simulink model "mpc_controller1"  (R2024a)
settings: Solver=VariableStepAuto  StartTime=0.0  StopTime=12  RelTol=1e-3
InitFcn:
  | % MPC Tuning:
  | % Control Voltage was low, settling of the state variables is slow.
  | % Sol1: Decrease mpc1.Weights.MVRate (the penalty on voltage be cheaper)
  | % Sol2: Increase the weights penalty (same, more expensive error)
  | % Sol3: Initial conditions should not be near the constraints.
  | 
  | % For 1000 Hz sample rate with sensors, and 100 Hz sample rate MPC, the
  | % 200 long predict and 10 long control horizon should be enough,
  | % the system can't change faster.
  | 
  | % MPC tuning params
  | horizonNum = 200;
  | controlHorizon = 10;
  | 
  | MVWeight = 0;
  | MVRateWeight = 0.1;
  | stateVariableWeights = [0 0 10 0 0 0];
  | ECR = 10;
  | 
  | % MPC Constraints
  | x_m = 0.1;
  | x_dot_m = 2;
  | phi_m = 0.2;
  | phi_dot_m = 5;
  | i_m = 2;
  | w_m = 100;
  | 
  | % Init model
  | dt = 1/1000;
  | model_dt = dt;
  | 
  | A_aug =[ 0    0.0010         0         0         0         0;
  |          0         0   -0.0010         0    0.8250         0;
  |          0         0         0    0.0010         0         0;
  |          0         0    0.0473         0   -3.6197         0;
  |          0         0         0         0   -0.0591   -0.0022;
  |          0         0         0         0    0.3401   -0.0031];
  | B_aug = [0
  |          0;
  |          0;
  |          0;
  |        200;
  |          0];
  | C_aug = [    1     0     0     0     0     0;
  |              0     0     1     0     0     0];
  | D_aug = [0;0];
  | 
  | % Discretize System - for the augmented system
  | sysd = c2d(ss(A_aug, B_aug, C_aug, 0), dt);
  | Ad_aug = sysd.A;
  | Bd_aug = sysd.B;
  | Cd_aug = sysd.C;
  | 
  | % MPC
  | mpc_dt = 1/100;
  | robSys_mpc = c2d(ss(A_aug, B_aug, eye(6), zeros(6,1)), mpc_dt);
  | %% create MPC controller object with sample time
  | mpc1 = mpc(robSys_mpc, mpc_dt);
  | %% specify prediction horizon
  | mpc1.PredictionHorizon = horizonNum;
  | %% specify control horizon
  | mpc1.ControlHorizon = controlHorizon;
  | %% specify nominal values for inputs and outputs
  | mpc1.Model.Nominal.U = 0;
  | mpc1.Model.Nominal.Y = [0;0;0;0;0;0];
  | %% specify constraints for MV and MV Rate
  | mpc1.MV(1).Min = -12;
  | mpc1.MV(1).Max = 12;
  | %% specify constraints for OV
  | mpc1.OV(1).Min = -x_m;
  | mpc1.OV(1).Max = x_m;
  | mpc1.OV(2).Min = -x_dot_m;
  | mpc1.OV(2).Max = x_dot_m;
  | mpc1.OV(3).Min = -phi_m;
  | mpc1.OV(3).Max = phi_m;
  | mpc1.OV(4).Min = -phi_dot_m;
  | mpc1.OV(4).Max = phi_dot_m;
  | mpc1.OV(5).Min = -i_m;
  | mpc1.OV(5).Max = i_m;
  | mpc1.OV(6).Min = -w_m;
  | mpc1.OV(6).Max = w_m;
  | %% specify overall adjustment factor applied to weights
  | beta = 6.821;
  | %% specify weights
  | mpc1.Weights.MV = MVWeight;
  | mpc1.Weights.MVRate = MVRateWeight;
  | mpc1.Weights.OV = stateVariableWeights;
  | mpc1.Weights.ECR = ECR;
  | %% specify overall adjustment factor applied to estimation model gains
  | alpha = 4.1687;
  | %% adjust default output disturbance model gains
  | setoutdist(mpc1, 'model', getoutdist(mpc1)*alpha);
  | %% adjust default measurement noise model gains
  | mpc1.Model.Noise = mpc1.Model.Noise/alpha;
  | %% specify simulation options
  | options = mpcsimopt();
  | options.RefLookAhead = 'off';
  | options.MDLookAhead = 'off';
  | options.Constraints = 'on';
  | options.OpenLoop = 'off';
undefined symbols (not defined in the file or in its folder): Discrete, Time
libraries: ctrlSharedLib x1, mpclib x1
settings Model: Creator=Peter  LastModifiedBy=Peter

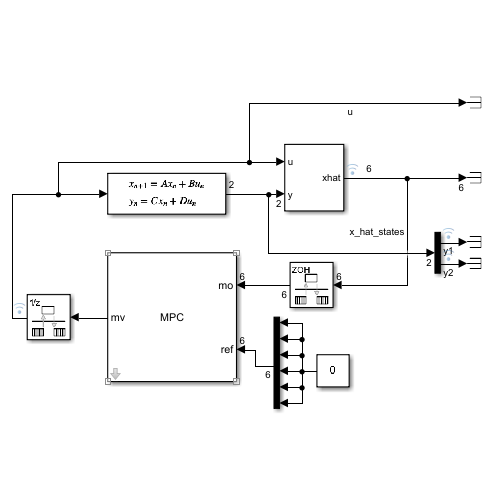
[thumbnail: Simulink's stored preview of the top-level diagram]
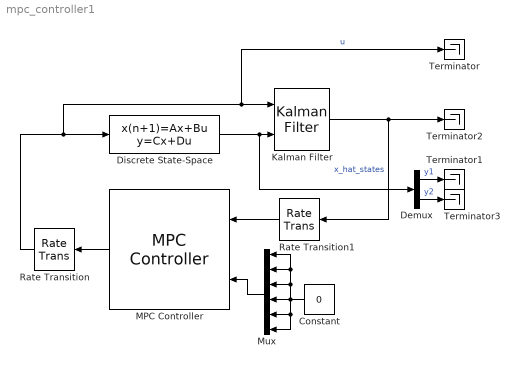
== system mpc_controller1 ==
  Constant : Constant  Value=0
  Demux : Demux  Outputs=2
  Discrete State-Space : DiscreteStateSpace  A=Ad_aug  B=Bd_aug  C=Cd_aug  D=[0;0]  InitialCondition=[0;0;0.05;0;0;0]  SampleTime=model_dt
  Kalman Filter : ctrlSharedLib/Kalman Filter  TimeDomain=Discrete-Time  UseCurrentEstimator=on  ModelSource=Individual A, B, C, D matrices  ModelSourceVariable=ss(0.95,1,1,0,1)  A=Ad_aug  B=Bd_aug  C=Cd_aug  D=[0;0]  NumberOfStates=1  NumberOfInputs=1  NumberOfOutputs=1  InitialEstimateSource=Dialog  X0=0  P0=10  UseK=off  UseGH=off  NumberOfProcessNoiseInputs=1  G=1  TimeInvariantG=on  H=0  TimeInvariantH=on  Q=diag(ones(1,6))*0.1  TimeInvariantQ=on  R=diag(ones(1,2))*0.1  TimeInvariantR=on  N=0  TimeInvariantN=on  AddInputPort=on  AddEnablePort=off  OutputEstimatedY=off  OutputP=off  Ts=model_dt
  MPC Controller : mpclib/MPC Controller  SCDEnableBlockLinearizationSpecification=on  mpcobj=mpc1  is_multiple=0  enable_value=0  return_u0=off  updateMPCinCallerWorkspace=on  md_inport=off  mv_inport=off  uref_inport=off  return_cost=off  return_mvseq=off  return_qpstatus=off  return_xseq=off  return_state=off  return_ovseq=off  state_inport=off  umin_inport=off  umax_inport=off  ymin_inport=off  ymax_inport=off  cc_inport=off  ywt_inport=off  uwt_inport=off  duwt_inport=off  rhoeps_inport=off  pm_inport=off  MaximumP=10  HorizonChoice=FixedHorizon  n_ts=0.01  n_p=200  n_mv=1  n_md=0  n_ud=0  n_mo=6  n_uo=0  BlockDataType=double  SampleTimeInherited=off  switch_inport=off
  Mux : Mux  Inputs=6
  Rate Transition : RateTransition
  Rate Transition1 : RateTransition
  Terminator{,1..3} (4 alike) : Terminator
  wires:
  Discrete State-Space/1 -> Demux/1, Kalman Filter/2
  Kalman Filter/1 -> Rate Transition1/1, Terminator2/1  "x_hat_states"
  MPC Controller/1 -> Rate Transition/1
  Mux/1 -> MPC Controller/2
  Constant/1 -> Mux/1, Mux/2, Mux/3, Mux/6, Mux/5, Mux/4
  Rate Transition/1 -> Terminator/1, Kalman Filter/1, Discrete State-Space/1  "u"
  Rate Transition1/1 -> MPC Controller/1
  Demux/1 -> Terminator1/1  "y1"
  Demux/2 -> Terminator3/1  "y2"
